simulink model "seven"  (R2015b)
settings: Solver=ode45  StartTime=0.0  StopTime=10  RelTol=1e-3
settings Model: Creator=朱明菲  LastModifiedBy=朱明菲

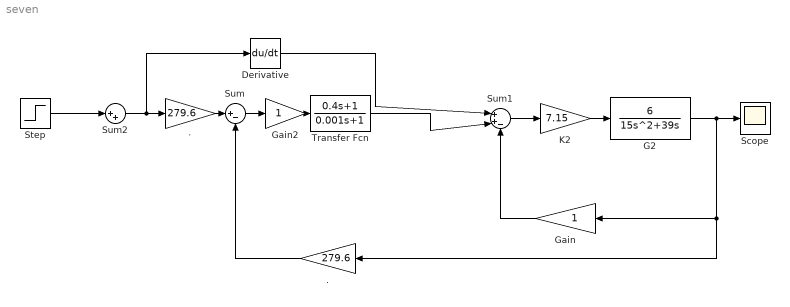
== system seven ==
  " ·" : Gain  Gain=279.6
  ". " : Gain  Gain=279.6
  Derivative : Derivative
  G2 : TransferFcn  Numerator=[6]  Denominator=[15 39 0]
  Gain : Gain
  Gain2 : Gain
  K2 : Gain  Gain=7.15
  Scope : Scope
  Step : Step  SampleTime=0
  Sum : Sum  Inputs=|+-
  Sum1 : Sum  Inputs=|++-
  Sum2 : Sum  Inputs=|++
  Transfer Fcn : TransferFcn  Numerator=[0.4 1]  Denominator=[0.001 1]
  wires:
  " ·"/1 -> Sum/1
  Sum/1 -> Gain2/1
  K2/1 -> G2/1
  ". "/1 -> Sum/2
  G2/1 -> Scope/1, Gain/1, ". "/1
  Gain/1 -> Sum1/3
  Derivative/1 -> Sum1/1
  Sum1/1 -> K2/1
  Step/1 -> Sum2/1
  Sum2/1 -> Derivative/1, " ·"/1
  Gain2/1 -> Transfer Fcn/1
  Transfer Fcn/1 -> Sum1/2
